simulink model "DSB_SC_Simulink"  (R2024b)
settings: Solver=VariableStepAuto  StartTime=0.0  StopTime=10.0  RelTol=1e-3
settings Model: Creator=LENOVO  LastModifiedBy=LENOVO

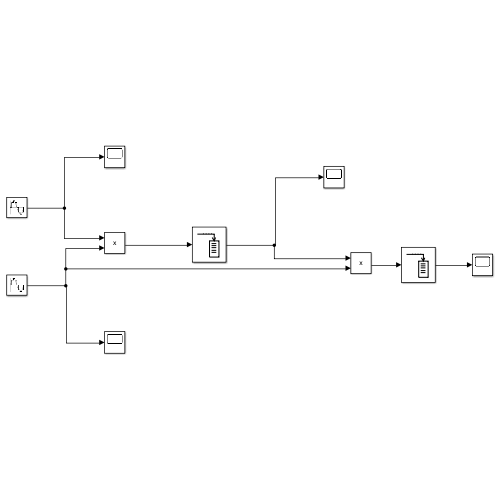
[thumbnail: Simulink's stored preview of the top-level diagram]
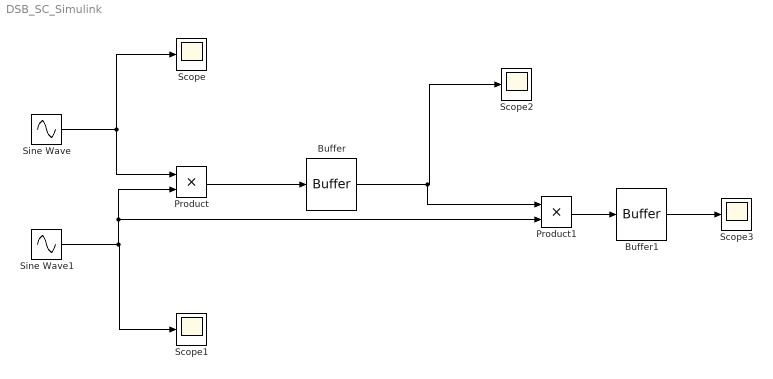
== system DSB_SC_Simulink ==
  Buffer : Buffer  OutputFrames=off
  Buffer1 : Buffer  OutputFrames=off
  Product : Product
  Product1 : Product
  Scope{,1..3} (4 alike) : Scope
  Sine Wave : Sin  Amplitude=2  SampleTime=0.001
  Sine Wave1 : Sin  Amplitude=2  Frequency=10  SampleTime=0.001
  wires:
  Sine Wave/1 -> Scope/1, Product/1
  Sine Wave1/1 -> Product1/2, Product/2, Scope1/1
  Product/1 -> Buffer/1
  Buffer/1 -> Product1/1, Scope2/1
  Product1/1 -> Buffer1/1
  Buffer1/1 -> Scope3/1
